simulink model "bipedal_robot_buV2_4"  (R2020b)
settings: Solver=ode23  StartTime=0.0  StopTime=Tsim  MaxStep=0.01  RelTol=1e-3  AbsTol=1e-3  EnableMultiTasking=on
undefined symbols (not defined in the file): Base, ctrl_config, ctrl_data, g, LefAnklePitch, LefAnkleRoll, LefHipPitch, LefHipRoll, LefHipYaw, LefKnee, lleg_str, RigAnklePitch, RigAnkleRoll, RigHipPitch, RigHipRoll, RigHipYaw, RigKnee, rleg_str, sim_floor, Tfil, TG_test_type, total_mass, Ts, X, Y, Z
libraries: sm_lib x53, biped_lib x34, nesl_utility x9, robotmaniplib x5, simulink x1, Contact_Forces_Lib x1
(part 2 of 3)

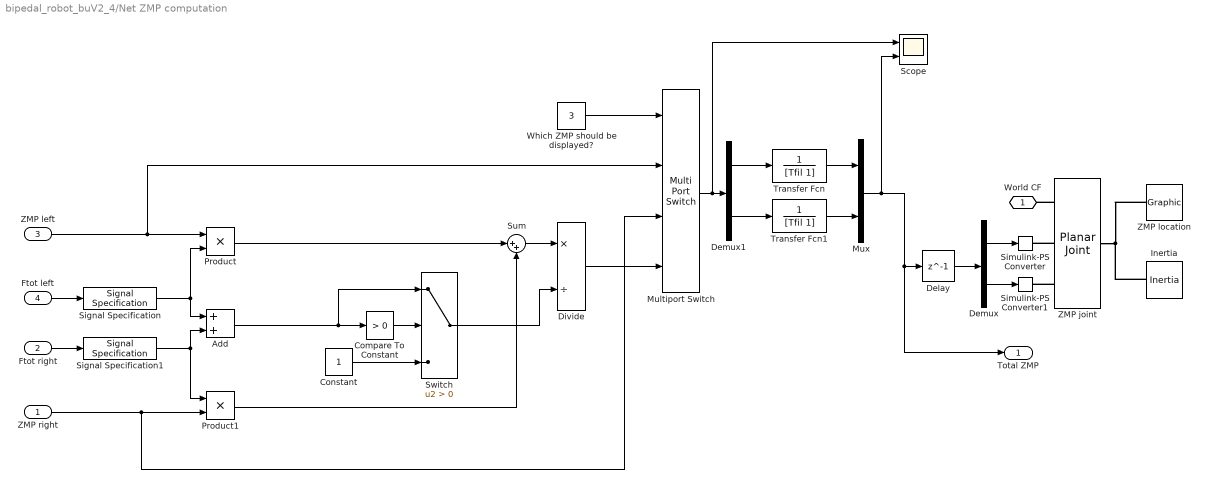
== system bipedal_robot_buV2_4/Net ZMP computation ==
  ZMP right : Inport
  Ftot right : Inport  Port=2
  ZMP left : Inport  Port=3
  Ftot left : Inport  Port=4
  Add : Sum
  Compare To Constant : simulink/Logic and Bit Operations/Compare To Constant  relop=>  const=0  OutDataTypeStr=boolean
  Constant : Constant
  Delay : Delay  DelayLength=1  InitialCondition=0  SampleTime=Ts/10
  Demux : Demux  Outputs=2
  Demux1 : Demux  Outputs=2
  Divide : Product  Inputs=*/
  Inertia : sm_lib/Body Elements/Inertia  InertiaType=Custom  Mass=10  MassUnits=g  CenterOfMass=[0 0 0]  CenterOfMassUnits=m  MomentsOfInertia=ones(3,1)*0.001  MomentsOfInertiaUnits=kg*m^2  ProductsOfInertia=[0 0 0]  ProductsOfInertiaUnits=kg*m^2  GraphicType=None  MarkerShape=Inertia  MarkerSize=20  GraphicVisPropType=SimpleVisualProperties  GraphicDiffuseColor=[0.5 0.5 0.5]  GraphicSpecularColor=[0.5 0.5 0.5 1.0]  GraphicAmbientColor=[0.15 0.15 0.15 1.0]  GraphicEmissiveColor=[0.0 0.0 0.0 1.0]  GraphicShininess=75  GraphicOpacity=1.0
  Multiport Switch : MultiPortSwitch
  Mux : Mux  Inputs=2
  Product : Product
  Product1 : Product
  Scope : Scope  NumInputPorts=2
  Signal Specification : SignalSpecification  Dimensions=1
  Signal Specification1 : SignalSpecification  Dimensions=1
  Simulink-PS Converter : nesl_utility/Simulink-PS Converter  PhysicalDomain=network_engine_domain  SubClassName=ps_input  LeftPortType=input  RightPortType=output  PseudoPeriodic=off  Frequencies=[]  NoiseDistribution=none  NoiseParameters=[]  Unit=1  AffineConversion=off  FilteringAndDerivatives=zero  SimscapeFilterOrder=1  InputFilterTimeConstant=0.001  UdotUserProvided=0
      settings: SourceProductName=Utilities
  Simulink-PS Converter1 : nesl_utility/Simulink-PS Converter  PhysicalDomain=network_engine_domain  SubClassName=ps_input  LeftPortType=input  RightPortType=output  PseudoPeriodic=off  Frequencies=[]  NoiseDistribution=none  NoiseParameters=[]  Unit=1  AffineConversion=off  FilteringAndDerivatives=zero  SimscapeFilterOrder=1  InputFilterTimeConstant=0.001  UdotUserProvided=0
      settings: SourceProductName=Utilities
  Sum : Sum  Inputs=|++
  Switch : Switch  Criteria=u2 > Threshold
  Transfer Fcn : TransferFcn  Denominator=[Tfil 1]
  Transfer Fcn1 : TransferFcn  Denominator=[Tfil 1]
  Which ZMP should be displayed? : Constant  Value=3
  ZMP joint : sm_lib/Joints/Planar Joint  JointMode=Normal  SenseConstraintForce=off  SenseConstraintForceX=off  SenseConstraintForceY=off  SenseConstraintForceZ=off  SenseConstraintTorque=off  SenseConstraintTorqueX=off  SenseConstraintTorqueY=off  SenseConstraintTorqueZ=off  SenseTotalForce=off  SenseTotalForceX=off  SenseTotalForceY=off  SenseTotalForceZ=off  SenseTotalTorque=off  SenseTotalTorqueX=off  SenseTotalTorqueY=off  SenseTotalTorqueZ=off  CompositeWrenchDir=FollowerOnBase  CompositeWrenchFrame=BaseFrame  PxEquilibriumPosition=0  PxEquilibriumPositionUnits=m  PxSpringStiffness=0  PxSpringStiffnessUnits=N/m  PxDampingCoefficient=0  PxDampingCoefficientUnits=N/(m/s)  PxTorqueActuationMode=ComputedTorque  PxMotionActuationMode=InputMotion  PxSensePosition=off  PxSenseVelocity=off  PxSenseAcceleration=off  PxSenseTorqueForce=off  PxSenseLowerLimitTorqueForce=off  PxSenseUpperLimitTorqueForce=off  PxLowerLimitSpecify=off  PxLowerLimitBound=-1  PxLowerLimitBoundUnits=m  PxLowerLimitStiffness=1e6  PxLowerLimitStiffnessUnits=N/m  PxLowerLimitDamping=1e3  PxLowerLimitDampingUnits=N/(m/s)  PxLowerLimitTransitionRegionWidth=1e-4  PxLowerLimitTransitionRegionWidthUnits=m  PxUpperLimitSpecify=off  PxUpperLimitBound=1  PxUpperLimitBoundUnits=m  PxUpperLimitStiffness=1e6  PxUpperLimitStiffnessUnits=N/m  PxUpperLimitDamping=1e3  PxUpperLimitDampingUnits=N/(m/s)  PxUpperLimitTransitionRegionWidth=1e-4  PxUpperLimitTransitionRegionWidthUnits=m  PxPositionTargetSpecify=off  PxPositionTargetPriority=High  PxPositionTargetValue=0  PxPositionTargetValueUnits=m  PxVelocityTargetSpecify=off  PxVelocityTargetPriority=High  PxVelocityTargetValue=0  PxVelocityTargetValueUnits=m/s  PyEquilibriumPosition=0  PyEquilibriumPositionUnits=m  PySpringStiffness=0  PySpringStiffnessUnits=N/m  PyDampingCoefficient=0  PyDampingCoefficientUnits=N/(m/s)  PyTorqueActuationMode=ComputedTorque  PyMotionActuationMode=InputMotion  PySensePosition=off  PySenseVelocity=off  PySenseAcceleration=off  PySenseTorqueForce=off  PySenseLowerLimitTorqueForce=off  PySenseUpperLimitTorqueForce=off  PyLowerLimitSpecify=off  PyLowerLimitBound=-1  PyLowerLimitBoundUnits=m  PyLowerLimitStiffness=1e6  PyLowerLimitStiffnessUnits=N/m  PyLowerLimitDamping=1e3  PyLowerLimitDampingUnits=N/(m/s)  PyLowerLimitTransitionRegionWidth=1e-4  PyLowerLimitTransitionRegionWidthUnits=m  PyUpperLimitSpecify=off  PyUpperLimitBound=1  PyUpperLimitBoundUnits=m  PyUpperLimitStiffness=1e6  PyUpperLimitStiffnessUnits=N/m  PyUpperLimitDamping=1e3  PyUpperLimitDampingUnits=N/(m/s)  PyUpperLimitTransitionRegionWidth=1e-4  PyUpperLimitTransitionRegionWidthUnits=m  PyPositionTargetSpecify=off  PyPositionTargetPriority=High  PyPositionTargetValue=0  PyPositionTargetValueUnits=m  PyVelocityTargetSpecify=off  PyVelocityTargetPriority=High  PyVelocityTargetValue=0  PyVelocityTargetValueUnits=m/s  RzEquilibriumPosition=0  RzEquilibriumPositionUnits=deg  RzSpringStiffness=0  RzSpringStiffnessUnits=N*m/deg  RzDampingCoefficient=0  RzDampingCoefficientUnits=N*m/(deg/s)  RzTorqueActuationMode=NoTorque  RzMotionActuationMode=ComputedMotion  RzSensePosition=off  RzSenseVelocity=off  RzSenseAcceleration=off  RzSenseTorqueForce=off  RzSenseLowerLimitTorqueForce=off  RzSenseUpperLimitTorqueForce=off  RzLowerLimitSpecify=off  RzLowerLimitBound=-90  RzLowerLimitBoundUnits=deg  RzLowerLimitStiffness=1e4  RzLowerLimitStiffnessUnits=N*m/deg  RzLowerLimitDamping=10  RzLowerLimitDampingUnits=N*m/(deg/s)  RzLowerLimitTransitionRegionWidth=0.1  RzLowerLimitTransitionRegionWidthUnits=deg  RzUpperLimitSpecify=off  RzUpperLimitBound=90  RzUpperLimitBoundUnits=deg  RzUpperLimitStiffness=1e4  RzUpperLimitStiffnessUnits=N*m/deg  RzUpperLimitDamping=10  RzUpperLimitDampingUnits=N*m/(deg/s)  RzUpperLimitTransitionRegionWidth=0.1  RzUpperLimitTransitionRegionWidthUnits=deg  RzPositionTargetSpecify=off  RzPositionTargetPriority=High  RzPositionTargetValue=0  RzPositionTargetValueUnits=deg  RzVelocityTargetSpecify=off  RzVelocityTargetPriority=High  RzVelocityTargetValue=0  RzVelocityTargetValueUnits=deg/s
  ZMP location : sm_lib/Body Elements/Graphic  GraphicType=Marker  MarkerShape=Frame  MarkerSize=30  GraphicVisPropType=SimpleVisualProperties  GraphicDiffuseColor=[0.0 1.0 0.2]  GraphicSpecularColor=[0.5 0.5 0.5 1.0]  GraphicAmbientColor=[0.15 0.15 0.15 1.0]  GraphicEmissiveColor=[0.0 0.0 0.0 1.0]  GraphicShininess=75  GraphicOpacity=1.0
  World CF : PMIOPort  Side=Left
  Total ZMP : Outport
  wires:
  ZMP left/1 -> Product/1, Multiport Switch/2
  Signal Specification/1 -> Product/2, Add/1
  Signal Specification1/1 -> Product1/1, Add/2
  ZMP right/1 -> Multiport Switch/3, Product1/2
  Product/1 -> Sum/1
  Product1/1 -> Sum/2
  Sum/1 -> Divide/1
  Add/1 -> Compare To Constant/1, Switch/1
  Mux/1 -> Total ZMP/1, Delay/1, Scope/2
  Demux/1 -> Simulink-PS Converter/1
  Demux/2 -> Simulink-PS Converter1/1
  Compare To Constant/1 -> Switch/2
  Constant/1 -> Switch/3
  Switch/1 -> Divide/2
  Ftot left/1 -> Signal Specification/1
  Ftot right/1 -> Signal Specification1/1
  Delay/1 -> Demux/1
  Which ZMP should be displayed?/1 -> Multiport Switch/1
  Divide/1 -> Multiport Switch/4
  Demux1/1 -> Transfer Fcn/1
  Demux1/2 -> Transfer Fcn1/1
  Multiport Switch/1 -> Scope/1, Demux1/1
  Transfer Fcn1/1 -> Mux/2
  Transfer Fcn/1 -> Mux/1
  connections:
  ZMP joint/LConn1 -- World CF/RConn1
  ZMP location/RConn1 -- Inertia/RConn1 -- ZMP joint/RConn1
  ZMP joint/LConn2 -- Simulink-PS Converter/RConn1
  ZMP joint/LConn3 -- Simulink-PS Converter1/RConn1

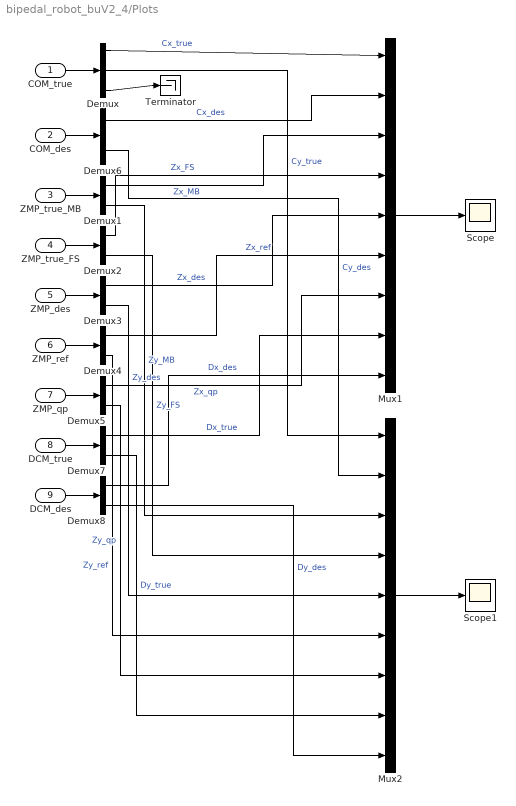
== system bipedal_robot_buV2_4/Plots ==
  COM_true : Inport
  COM_des : Inport  Port=2
  ZMP_true_MB : Inport  Port=3
  ZMP_true_FS : Inport  Port=4
  ZMP_des : Inport  Port=5
  ZMP_ref : Inport  Port=6
  ZMP_qp : Inport  Port=7
  DCM_true : Inport  Port=8
  DCM_des : Inport  Port=9
  Demux : Demux  Outputs=3
  Demux{1..8} (8 alike) : Demux  Outputs=2
  Mux1 : Mux  Inputs=9
  Mux2 : Mux  Inputs=9
  Scope : Scope
  Scope1 : Scope
  Terminator : Terminator
  wires:
  ZMP_true_MB/1 -> Demux1/1
  ZMP_true_FS/1 -> Demux2/1
  ZMP_des/1 -> Demux3/1
  ZMP_ref/1 -> Demux4/1
  ZMP_qp/1 -> Demux5/1
  COM_true/1 -> Demux/1
  DCM_true/1 -> Demux7/1
  DCM_des/1 -> Demux8/1
  Demux/1 -> Mux1/1  "Cx_true"
  Demux6/1 -> Mux1/2  "Cx_des"
  Demux1/1 -> Mux1/3  "Zx_MB"
  Demux2/1 -> Mux1/4  "Zx_FS"
  Demux3/1 -> Mux1/5  "Zx_des"
  Demux4/1 -> Mux1/6  "Zx_ref"
  Demux5/1 -> Mux1/7  "Zx_qp"
  Demux7/1 -> Mux1/8  "Dx_true"
  Demux8/1 -> Mux1/9  "Dx_des"
  Demux/2 -> Mux2/1  "Cy_true"
  Demux1/2 -> Mux2/3  "Zy_MB"
  Demux2/2 -> Mux2/4  "Zy_FS"
  Demux3/2 -> Mux2/5  "Zy_des"
  Demux4/2 -> Mux2/6  "Zy_ref"
  Demux5/2 -> Mux2/7  "Zy_qp"
  Demux7/2 -> Mux2/8  "Dy_true"
  Demux8/2 -> Mux2/9  "Dy_des"
  Demux6/2 -> Mux2/2  "Cy_des"
  Demux/3 -> Terminator/1
  Mux1/1 -> Scope/1
  Mux2/1 -> Scope1/1
  COM_des/1 -> Demux6/1

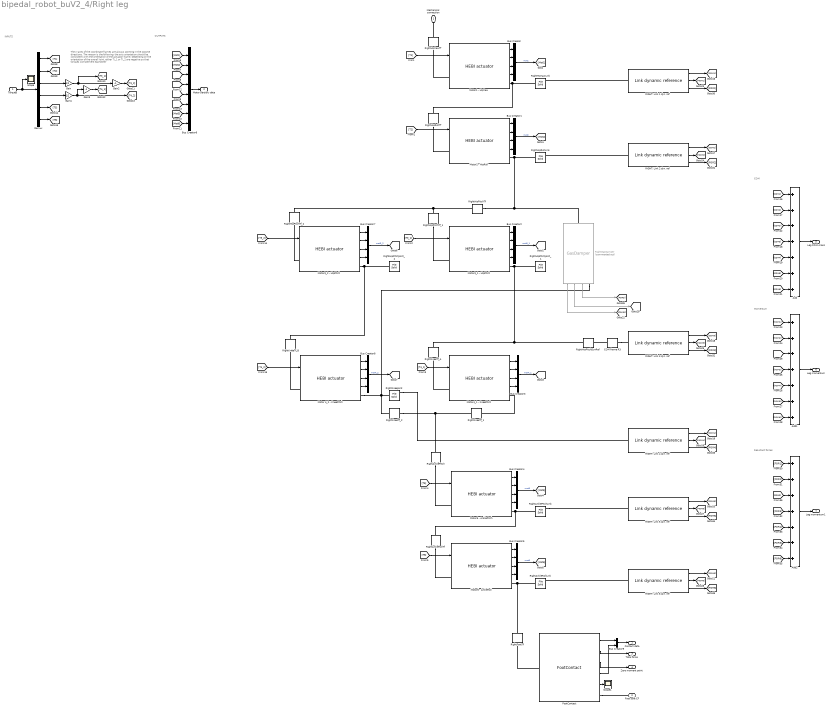
== system bipedal_robot_buV2_4/Right leg ==
  note: OUTPUTS
  note: INPUTS
  note: The z-axes of the coordinate frames are always pointing in the
      | oposite directions. The reason is the following: the axis orientation
      | should be consistent with the orientation of the actuator frame. Depending on the orientation of the overall joint, either Ti_1 or Ti_2
      | are negative so that torques complement eachother
  note: Resultant forces
  note: Momentum
  note: COM
  Torques : Inport
  Add : Sum  Inputs=7
  Add1 : Sum  Inputs=7
  Add2 : Sum  Inputs=7
  Bus Creator{,1..5,7..8} (8 alike) : BusCreator  Inputs=4
  Bus Creator6 : BusCreator  Inputs=8  OutDataTypeStr=Bus: leg_str_bus
  Bus Creator9 : BusCreator  Inputs=2
  COM frame R3 : sm_lib/Frames and Transforms/Rigid Transform  TranslationMethod=Cartesian  TranslationStandardOffset=0  TranslationLengthUnit=m  TranslationStandardAxis=+Z  TranslationCartesianOffset=RigHipPitch.body.com  TranslationROffset=0  TranslationROffsetUnits=m  TranslationZOffset=0  TranslationZOffsetUnits=m  TranslationThetaOffset=0  TranslationThetaOffsetUnits=deg  RotationMethod=None  RotationAngleUnits=deg  RotationStandardAxis=+Z  RotationAngle=0.0  RotationArbitraryAxis=[0 0 1]  FollAlignAxisA=+X  BaseAlignAxisA=+Y  FollAlignAxisB=+Y  BaseAlignAxisB=+Z  RotationSequenceAxes=FollowerAxes  RotationSequence=XYX  RotationSequenceAngles=[0 0 0]  RotationSequenceAnglesUnits=deg  RotationMatrix=[1 0 0; 0 1 0; 0 0 1]
  Demux : Demux  Outputs=6
  FootContact : biped_lib/FootContact  SystemSampleTime=-1  VariantActivationTime=update diagram  Latency=0  AutoFrameSizeCalculation=off
  Gain : Gain  Gain=1/2
  Gain1 : Gain  Gain=1/2
  Gain2 : Gain  Gain=-1
  Gain3 : Gain  Gain=-1
  Motor 4_2 - KneePitch : biped_lib/HEBI actuator  Tmax=motor.X8.v16.Tmax  qinit=RigKnee.qinit_2  IMU=RigKnee.IMU_2
  Motor1 - HipYaw : biped_lib/HEBI actuator  Tmax=motor.X8.v16.Tmax  qinit=RigHipYaw.qinit  IMU=RigHipYaw.IMU
  Motor2 - HipRoll : biped_lib/HEBI actuator  Tmax=motor.X8.v16.Tmax  qinit=RigHipRoll.qinit  IMU=RigHipRoll.IMU
  Motor3_1 - HipPitch : biped_lib/HEBI actuator  Tmax=motor.X8.v16.Tmax  qinit=RigHipPitch.qinit_1  IMU=RigHipPitch.IMU_1
  Motor3_2 - HipPitch : biped_lib/HEBI actuator  Tmax=motor.X8.v16.Tmax  qinit=RigHipPitch.qinit_2  IMU=RigHipPitch.IMU_2
  Motor4_1 - KneePitch : biped_lib/HEBI actuator  Tmax=motor.X8.v16.Tmax  qinit=RigKnee.qinit_1  IMU=RigKnee.IMU_1
  Motor5 - AnklePitch : biped_lib/HEBI actuator  Tmax=motor.X8.v16.Tmax  qinit=RigAnklePitch.qinit  IMU=RigAnklePitch.IMU
  Motor6 - AnkleRoll : biped_lib/HEBI actuator  Tmax=motor.X8.v16.Tmax  qinit=RigAnkleRoll.qinit  IMU=RigAnkleRoll.IMU
  RIGHT: Link 1 dyn. ref : biped_lib/Link dynamic reference  M=RigHipYaw.body.mass  I=RigHipYaw.body.inertia
  RIGHT: Link 2 dyn. ref : biped_lib/Link dynamic reference  M=RigHipRoll.body.mass  I=RigHipRoll.body.inertia
  RIGHT: Link 3 dyn. ref : biped_lib/Link dynamic reference  M=RigHipPitch.body.mass  I=RigHipPitch.body.inertia
  RIGHT: Link 4 dyn. ref : biped_lib/Link dynamic reference  M=RigKnee.body.mass  I=RigKnee.body.inertia
  RIGHT: Link 5 dyn. ref : biped_lib/Link dynamic reference  M=RigAnklePitch.body.mass  I=RigAnklePitch.body.inertia
  RIGHT: Link 6 dyn. ref : biped_lib/Link dynamic reference  M=RigAnkleRoll.body.mass  I=RigAnkleRoll.body.inertia
  RightAnklePitch : sm_lib/Frames and Transforms/Rigid Transform  TranslationMethod=Cartesian  TranslationStandardOffset=0  TranslationLengthUnit=m  TranslationStandardAxis=+Z  TranslationCartesianOffset=RigAnklePitch.pos  TranslationROffset=0  TranslationROffsetUnits=m  TranslationZOffset=0  TranslationZOffsetUnits=m  TranslationThetaOffset=0  TranslationThetaOffsetUnits=deg  RotationMethod=RotationSequence  RotationAngleUnits=deg  RotationStandardAxis=+Z  RotationAngle=0.0  RotationArbitraryAxis=[0 0 1]  FollAlignAxisA=+X  BaseAlignAxisA=+Y  FollAlignAxisB=+Y  BaseAlignAxisB=+Z  RotationSequenceAxes=FollowerAxes  RotationSequence=XYZ  RotationSequenceAngles=RigAnklePitch.rot  RotationSequenceAnglesUnits=rad  RotationMatrix=[1 0 0; 0 1 0; 0 0 1]
  RightAnklePitchLink : sm_lib/Body Elements/File Solid  ExtGeomFileName=Link5R_LR.stl  UnitType=Custom  ExtGeomFileUnits=mm  StepReaderType=HEX  ExportConvexHullGeometry=on  InertiaType=CalculateFromGeometry  Mass=RigAnklePitch.body.mass  MassUnits=kg  CenterOfMass=[0 0 0]  CenterOfMassUnits=m  MomentsOfInertia=[1 1 1]  MomentsOfInertiaUnits=kg*m^2  ProductsOfInertia=[0 0 0]  ProductsOfInertiaUnits=kg*m^2  BasedOnType=Mass  Density=1000  DensityUnits=kg/m^3  DoExposeReferenceFrame=on  SerializedFrames=<Frames><Frame><Id>Frame1</Id><Value><Name>COM</Name><Origin><Source>CenterOfMassFrame</Source><FeatureName></FeatureName></Origin><PrimaryAxis><DefinedDirection>+Z</DefinedDirection><Source>ReferenceFrame</Source><SourceDirection>+Z</SourceDirection><FeatureName></FeatureName></PrimaryAxis><SecondaryAxis><DefinedDirection>+X</DefinedDirection><Source>ReferenceFrame</Source><SourceDirection>+X</SourceDirection><FeatureName></FeatureName></SecondaryAxis></Value></Frame></Frames>  GraphicType=FromGeometry  MarkerShape=Sphere  MarkerSize=10  GraphicVisPropType=SimpleVisualProperties  GraphicDiffuseColor=[0.5 0.5 0.5]  GraphicSpecularColor=[0.5 0.5 0.5 1.0]  GraphicAmbientColor=[0.15 0.15 0.15 1.0]  GraphicEmissiveColor=[0.0 0.0 0.0 1.0]  GraphicShininess=75  GraphicOpacity=1.0
  RightAnkleRollLink : sm_lib/Body Elements/File Solid  ExtGeomFileName=Link6_LR.stl  UnitType=Custom  ExtGeomFileUnits=mm  StepReaderType=HEX  ExportConvexHullGeometry=on  InertiaType=CalculateFromGeometry  Mass=RigAnkleRoll.body.mass  MassUnits=kg  CenterOfMass=[0 0 0]  CenterOfMassUnits=m  MomentsOfInertia=[1 1 1]  MomentsOfInertiaUnits=kg*m^2  ProductsOfInertia=[0 0 0]  ProductsOfInertiaUnits=kg*m^2  BasedOnType=Mass  Density=1000  DensityUnits=kg/m^3  DoExposeReferenceFrame=on  SerializedFrames=<Frames><Frame><Id>Frame1</Id><Value><Name>COM</Name><Origin><Source>CenterOfMassFrame</Source><FeatureName></FeatureName></Origin><PrimaryAxis><DefinedDirection>+Z</DefinedDirection><Source>ReferenceFrame</Source><SourceDirection>+Z</SourceDirection><FeatureName></FeatureName></PrimaryAxis><SecondaryAxis><DefinedDirection>+X</DefinedDirection><Source>ReferenceFrame</Source><SourceDirection>+X</SourceDirection><FeatureName></FeatureName></SecondaryAxis></Value></Frame></Frames>  GraphicType=FromGeometry  MarkerShape=Sphere  MarkerSize=10  GraphicVisPropType=SimpleVisualProperties  GraphicDiffuseColor=[0.5 0.5 0.5]  GraphicSpecularColor=[0.5 0.5 0.5 1.0]  GraphicAmbientColor=[0.15 0.15 0.15 1.0]  GraphicEmissiveColor=[0.0 0.0 0.0 1.0]  GraphicShininess=75  GraphicOpacity=1.0
  RightAnkleRollTf : sm_lib/Frames and Transforms/Rigid Transform  TranslationMethod=Cartesian  TranslationStandardOffset=0  TranslationLengthUnit=m  TranslationStandardAxis=+Z  TranslationCartesianOffset=RigAnkleRoll.pos  TranslationROffset=0  TranslationROffsetUnits=m  TranslationZOffset=0  TranslationZOffsetUnits=m  TranslationThetaOffset=0  TranslationThetaOffsetUnits=deg  RotationMethod=RotationSequence  RotationAngleUnits=deg  RotationStandardAxis=+Z  RotationAngle=0.0  RotationArbitraryAxis=[0 0 1]  FollAlignAxisA=+Z  BaseAlignAxisA=+X  FollAlignAxisB=+Y  BaseAlignAxisB=+Y  RotationSequenceAxes=FollowerAxes  RotationSequence=XYZ  RotationSequenceAngles=RigAnkleRoll.rot  RotationSequenceAnglesUnits=rad  RotationMatrix=[1 0 0; 0 1 0; 0 0 1]
  RightFootTf : sm_lib/Frames and Transforms/Rigid Transform  TranslationMethod=Cartesian  TranslationStandardOffset=0  TranslationLengthUnit=m  TranslationStandardAxis=+Z  TranslationCartesianOffset=RigFoot.pos  TranslationROffset=0  TranslationROffsetUnits=m  TranslationZOffset=0  TranslationZOffsetUnits=m  TranslationThetaOffset=0  TranslationThetaOffsetUnits=deg  RotationMethod=RotationSequence  RotationAngleUnits=deg  RotationStandardAxis=+Z  RotationAngle=0.0  RotationArbitraryAxis=[0 0 1]  FollAlignAxisA=+Z  BaseAlignAxisA=+Y  FollAlignAxisB=+X  BaseAlignAxisB=+X  RotationSequenceAxes=FollowerAxes  RotationSequence=XYZ  RotationSequenceAngles=RigFoot.rot  RotationSequenceAnglesUnits=rad  RotationMatrix=[1 0 0; 0 1 0; 0 0 1]
  RightGasDamper : biped_lib/GasDamper  Commented=on  mech=RigDamper
  RightHipPitchDynRef : sm_lib/Frames and Transforms/Rigid Transform  TranslationMethod=Cartesian  TranslationStandardOffset=0  TranslationLengthUnit=m  TranslationStandardAxis=+Z  TranslationCartesianOffset=-RigHipPitch.pos_1  TranslationROffset=0  TranslationROffsetUnits=m  TranslationZOffset=0  TranslationZOffsetUnits=m  TranslationThetaOffset=0  TranslationThetaOffsetUnits=deg  RotationMethod=None  RotationAngleUnits=deg  RotationStandardAxis=+Z  RotationAngle=0.0  RotationArbitraryAxis=[0 0 1]  FollAlignAxisA=+X  BaseAlignAxisA=+Y  FollAlignAxisB=+Y  BaseAlignAxisB=+Z  RotationSequenceAxes=FollowerAxes  RotationSequence=XYX  RotationSequenceAngles=[0 0 0]  RotationSequenceAnglesUnits=deg  RotationMatrix=[1 0 0; 0 1 0; 0 0 1]
  RightHipPitchJoint_1 : sm_lib/Body Elements/File Solid  ExtGeomFileName=Link3_LR.stl  UnitType=Custom  ExtGeomFileUnits=mm  StepReaderType=HEX  ExportConvexHullGeometry=on  InertiaType=CalculateFromGeometry  Mass=RigHipPitch.body.mass  MassUnits=kg  CenterOfMass=[0 0 0]  CenterOfMassUnits=m  MomentsOfInertia=[1 1 1]  MomentsOfInertiaUnits=kg*m^2  ProductsOfInertia=[0 0 0]  ProductsOfInertiaUnits=kg*m^2  BasedOnType=Mass  Density=1000  DensityUnits=kg/m^3  DoExposeReferenceFrame=on  SerializedFrames=<Frames/>  GraphicType=FromGeometry  MarkerShape=Sphere  MarkerSize=10  GraphicVisPropType=SimpleVisualProperties  GraphicDiffuseColor=[0.5 0.5 0.5]  GraphicSpecularColor=[0.5 0.5 0.5 1.0]  GraphicAmbientColor=[0.15 0.15 0.15 1.0]  GraphicEmissiveColor=[0.0 0.0 0.0 1.0]  GraphicShininess=75  GraphicOpacity=1.0
  RightHipPitchJoint_2 : sm_lib/Body Elements/File Solid  ExtGeomFileName=Link3_LR.stl  UnitType=Custom  ExtGeomFileUnits=mm  StepReaderType=HEX  ExportConvexHullGeometry=on  InertiaType=CalculateFromGeometry  Mass=RigHipPitch.body.mass  MassUnits=kg  CenterOfMass=[0 0 0]  CenterOfMassUnits=m  MomentsOfInertia=[1 1 1]  MomentsOfInertiaUnits=kg*m^2  ProductsOfInertia=[0 0 0]  ProductsOfInertiaUnits=kg*m^2  BasedOnType=Mass  Density=1000  DensityUnits=kg/m^3  DoExposeReferenceFrame=on  SerializedFrames=<Frames/>  GraphicType=FromGeometry  MarkerShape=Sphere  MarkerSize=10  GraphicVisPropType=SimpleVisualProperties  GraphicDiffuseColor=[0.5 0.5 0.5]  GraphicSpecularColor=[0.5 0.5 0.5 1.0]  GraphicAmbientColor=[0.15 0.15 0.15 1.0]  GraphicEmissiveColor=[0.0 0.0 0.0 1.0]  GraphicShininess=75  GraphicOpacity=1.0
  RightHipPitchTf : sm_lib/Frames and Transforms/Rigid Transform  TranslationMethod=Cartesian  TranslationStandardOffset=0  TranslationLengthUnit=m  TranslationStandardAxis=+Z  TranslationCartesianOffset=RigHipPitch.pos  TranslationROffset=0  TranslationROffsetUnits=m  TranslationZOffset=0  TranslationZOffsetUnits=m  TranslationThetaOffset=0  TranslationThetaOffsetUnits=deg  RotationMethod=RotationSequence  RotationAngleUnits=deg  RotationStandardAxis=+Z  RotationAngle=0.0  RotationArbitraryAxis=[0 0 1]  FollAlignAxisA=+Z  BaseAlignAxisA=-X  FollAlignAxisB=+Y  BaseAlignAxisB=+Y  RotationSequenceAxes=FollowerAxes  RotationSequence=XYX  RotationSequenceAngles=RigHipPitch.rot  RotationSequenceAnglesUnits=rad  RotationMatrix=[1 0 0; 0 1 0; 0 0 1]
  RightHipPitchTf_1 : sm_lib/Frames and Transforms/Rigid Transform  TranslationMethod=Cartesian  TranslationStandardOffset=0  TranslationLengthUnit=m  TranslationStandardAxis=+Z  TranslationCartesianOffset=RigHipPitch.pos_1  TranslationROffset=0  TranslationROffsetUnits=m  TranslationZOffset=0  TranslationZOffsetUnits=m  TranslationThetaOffset=0  TranslationThetaOffsetUnits=deg  RotationMethod=RotationSequence  RotationAngleUnits=deg  RotationStandardAxis=+Z  RotationAngle=0.0  RotationArbitraryAxis=[0 0 1]  FollAlignAxisA=+X  BaseAlignAxisA=+Y  FollAlignAxisB=+Y  BaseAlignAxisB=+Z  RotationSequenceAxes=FollowerAxes  RotationSequence=XYZ  RotationSequenceAngles=RigHipPitch.rot_1  RotationSequenceAnglesUnits=rad  RotationMatrix=[1 0 0; 0 1 0; 0 0 1]
  RightHipPitchTf_2 : sm_lib/Frames and Transforms/Rigid Transform  TranslationMethod=Cartesian  TranslationStandardOffset=0  TranslationLengthUnit=m  TranslationStandardAxis=+Z  TranslationCartesianOffset=RigHipPitch.pos_2  TranslationROffset=0  TranslationROffsetUnits=m  TranslationZOffset=0  TranslationZOffsetUnits=m  TranslationThetaOffset=0  TranslationThetaOffsetUnits=deg  RotationMethod=RotationSequence  RotationAngleUnits=deg  RotationStandardAxis=+Z  RotationAngle=0.0  RotationArbitraryAxis=[0 0 1]  FollAlignAxisA=+X  BaseAlignAxisA=+Y  FollAlignAxisB=+Y  BaseAlignAxisB=+Z  RotationSequenceAxes=FollowerAxes  RotationSequence=XYZ  RotationSequenceAngles=RigHipPitch.rot_2  RotationSequenceAnglesUnits=rad  RotationMatrix=[1 0 0; 0 1 0; 0 0 1]
  RightHipRollLink : sm_lib/Body Elements/File Solid  ExtGeomFileName=Link2_LR.stl  UnitType=Custom  ExtGeomFileUnits=mm  StepReaderType=HEX  ExportConvexHullGeometry=on  InertiaType=CalculateFromGeometry  Mass=RigHipRoll.body.mass  MassUnits=kg  CenterOfMass=[0 0 0]  CenterOfMassUnits=m  MomentsOfInertia=[1 1 1]  MomentsOfInertiaUnits=kg*m^2  ProductsOfInertia=[0 0 0]  ProductsOfInertiaUnits=kg*m^2  BasedOnType=Mass  Density=1000  DensityUnits=kg/m^3  DoExposeReferenceFrame=on  SerializedFrames=<Frames><Frame><Id>Frame1</Id><Value><Name>COM</Name><Origin><Source>CenterOfMassFrame</Source><FeatureName></FeatureName></Origin><PrimaryAxis><DefinedDirection>+Z</DefinedDirection><Source>ReferenceFrame</Source><SourceDirection>+Z</SourceDirection><FeatureName></FeatureName></PrimaryAxis><SecondaryAxis><DefinedDirection>+X</DefinedDirection><Source>ReferenceFrame</Source><SourceDirection>+X</SourceDirection><FeatureName></FeatureName></SecondaryAxis></Value></Frame></Frames>  GraphicType=FromGeometry  MarkerShape=Sphere  MarkerSize=10  GraphicVisPropType=SimpleVisualProperties  GraphicDiffuseColor=[0.5 0.5 0.5]  GraphicSpecularColor=[0.5 0.5 0.5 1.0]  GraphicAmbientColor=[0.15 0.15 0.15 1.0]  GraphicEmissiveColor=[0.0 0.0 0.0 1.0]  GraphicShininess=75  GraphicOpacity=1.0
  RightHipRollTf : sm_lib/Frames and Transforms/Rigid Transform  TranslationMethod=Cartesian  TranslationStandardOffset=0  TranslationLengthUnit=m  TranslationStandardAxis=+Z  TranslationCartesianOffset=RigHipRoll.pos  TranslationROffset=0  TranslationROffsetUnits=m  TranslationZOffset=0  TranslationZOffsetUnits=m  TranslationThetaOffset=0  TranslationThetaOffsetUnits=deg  RotationMethod=RotationSequence  RotationAngleUnits=deg  RotationStandardAxis=+Z  RotationAngle=0.0  RotationArbitraryAxis=[0 0 1]  FollAlignAxisA=+Z  BaseAlignAxisA=+Y  FollAlignAxisB=+X  BaseAlignAxisB=+X  RotationSequenceAxes=FollowerAxes  RotationSequence=XYZ  RotationSequenceAngles=RigHipRoll.rot  RotationSequenceAnglesUnits=rad  RotationMatrix=[1 0 0; 0 1 0; 0 0 1]
  RightHipYawLink : sm_lib/Body Elements/File Solid  ExtGeomFileName=Link1R_LR.stl  UnitType=Custom  ExtGeomFileUnits=mm  StepReaderType=HEX  ExportConvexHullGeometry=on  InertiaType=CalculateFromGeometry  Mass=RigHipYaw.body.mass  MassUnits=kg  CenterOfMass=[0 0 0]  CenterOfMassUnits=m  MomentsOfInertia=[1 1 1]  MomentsOfInertiaUnits=kg*m^2  ProductsOfInertia=[0 0 0]  ProductsOfInertiaUnits=kg*m^2  BasedOnType=Mass  Density=1000  DensityUnits=kg/m^3  DoExposeReferenceFrame=on  SerializedFrames=<Frames><Frame><Id>Frame1</Id><Value><Name>COM</Name><Origin><Source>CenterOfMassFrame</Source><FeatureName></FeatureName></Origin><PrimaryAxis><DefinedDirection>+Z</DefinedDirection><Source>ReferenceFrame</Source><SourceDirection>+Z</SourceDirection><FeatureName></FeatureName></PrimaryAxis><SecondaryAxis><DefinedDirection>+X</DefinedDirection><Source>ReferenceFrame</Source><SourceDirection>+X</SourceDirection><FeatureName></FeatureName></SecondaryAxis></Value></Frame></Frames>  GraphicType=FromGeometry  MarkerShape=Sphere  MarkerSize=10  GraphicVisPropType=SimpleVisualProperties  GraphicDiffuseColor=[0.5 0.5 0.5]  GraphicSpecularColor=[0.5 0.5 0.5 1.0]  GraphicAmbientColor=[0.15 0.15 0.15 1.0]  GraphicEmissiveColor=[0.0 0.0 0.0 1.0]  GraphicShininess=75  GraphicOpacity=1.0
  RightHipYawTf : sm_lib/Frames and Transforms/Rigid Transform  TranslationMethod=Cartesian  TranslationStandardOffset=0  TranslationLengthUnit=m  TranslationStandardAxis=+Z  TranslationCartesianOffset=RigHipYaw.pos  TranslationROffset=0  TranslationROffsetUnits=m  TranslationZOffset=0  TranslationZOffsetUnits=m  TranslationThetaOffset=0  TranslationThetaOffsetUnits=deg  RotationMethod=RotationSequence  RotationAngleUnits=deg  RotationStandardAxis=+Z  RotationAngle=0.0  RotationArbitraryAxis=[0 0 1]  FollAlignAxisA=+X  BaseAlignAxisA=+Y  FollAlignAxisB=+Y  BaseAlignAxisB=+Z  RotationSequenceAxes=FollowerAxes  RotationSequence=XYZ  RotationSequenceAngles=RigHipYaw.rot  RotationSequenceAnglesUnits=rad  RotationMatrix=[1 0 0; 0 1 0; 0 0 1]
  RightKneeJoint : sm_lib/Body Elements/File Solid  ExtGeomFileName=Link4_LR.stl  UnitType=Custom  ExtGeomFileUnits=mm  StepReaderType=HEX  ExportConvexHullGeometry=on  InertiaType=CalculateFromGeometry  Mass=LefKnee.body.mass  MassUnits=kg  CenterOfMass=[0 0 0]  CenterOfMassUnits=m  MomentsOfInertia=[1 1 1]  MomentsOfInertiaUnits=kg*m^2  ProductsOfInertia=[0 0 0]  ProductsOfInertiaUnits=kg*m^2  BasedOnType=Mass  Density=1000  DensityUnits=kg/m^3  DoExposeReferenceFrame=on  SerializedFrames=<Frames><Frame><Id>Frame1</Id><Value><Name>COM</Name><Origin><Source>CenterOfMassFrame</Source><FeatureName></FeatureName></Origin><PrimaryAxis><DefinedDirection>+Z</DefinedDirection><Source>ReferenceFrame</Source><SourceDirection>+Z</SourceDirection><FeatureName></FeatureName></PrimaryAxis><SecondaryAxis><DefinedDirection>+X</DefinedDirection><Source>ReferenceFrame</Source><SourceDirection>+X</SourceDirection><FeatureName></FeatureName></SecondaryAxis></Value></Frame></Frames>  GraphicType=FromGeometry  MarkerShape=Sphere  MarkerSize=10  GraphicVisPropType=SimpleVisualProperties  GraphicDiffuseColor=[0.5 0.5 0.5]  GraphicSpecularColor=[0.5 0.5 0.5 1.0]  GraphicAmbientColor=[0.15 0.15 0.15 1.0]  GraphicEmissiveColor=[0.0 0.0 0.0 1.0]  GraphicShininess=75  GraphicOpacity=1.0
  RightKneeTf_1 : sm_lib/Frames and Transforms/Rigid Transform  TranslationMethod=Cartesian  TranslationStandardOffset=0  TranslationLengthUnit=m  TranslationStandardAxis=+Z  TranslationCartesianOffset=RigKnee.pos_1  TranslationROffset=0  TranslationROffsetUnits=m  TranslationZOffset=0  TranslationZOffsetUnits=m  TranslationThetaOffset=0  TranslationThetaOffsetUnits=deg  RotationMethod=RotationSequence  RotationAngleUnits=deg  RotationStandardAxis=+Z  RotationAngle=0.0  RotationArbitraryAxis=[0 0 1]  FollAlignAxisA=+X  BaseAlignAxisA=+Y  FollAlignAxisB=+Y  BaseAlignAxisB=+Z  RotationSequenceAxes=FollowerAxes  RotationSequence=XYZ  RotationSequenceAngles=RigKnee.rot_1  RotationSequenceAnglesUnits=rad  RotationMatrix=[1 0 0; 0 1 0; 0 0 1]
  RightKneeTf_2 : sm_lib/Frames and Transforms/Rigid Transform  TranslationMethod=Cartesian  TranslationStandardOffset=0  TranslationLengthUnit=m  TranslationStandardAxis=+Z  TranslationCartesianOffset=RigKnee.pos_2  TranslationROffset=0  TranslationROffsetUnits=m  TranslationZOffset=0  TranslationZOffsetUnits=m  TranslationThetaOffset=0  TranslationThetaOffsetUnits=deg  RotationMethod=RotationSequence  RotationAngleUnits=deg  RotationStandardAxis=+Z  RotationAngle=0.0  RotationArbitraryAxis=[0 0 1]  FollAlignAxisA=+X  BaseAlignAxisA=+Y  FollAlignAxisB=+Y  BaseAlignAxisB=+Z  RotationSequenceAxes=FollowerAxes  RotationSequence=XYZ  RotationSequenceAngles=RigKnee.rot_2  RotationSequenceAnglesUnits=rad  RotationMatrix=[1 0 0; 0 1 0; 0 0 1]
  RightKneeTf_A : sm_lib/Frames and Transforms/Rigid Transform  TranslationMethod=Cartesian  TranslationStandardOffset=0  TranslationLengthUnit=m  TranslationStandardAxis=+Z  TranslationCartesianOffset=RigKnee.pos  TranslationROffset=0  TranslationROffsetUnits=m  TranslationZOffset=0  TranslationZOffsetUnits=m  TranslationThetaOffset=0  TranslationThetaOffsetUnits=deg  RotationMethod=RotationSequence  RotationAngleUnits=deg  RotationStandardAxis=+Z  RotationAngle=0.0  RotationArbitraryAxis=[0 0 1]  FollAlignAxisA=+X  BaseAlignAxisA=+Y  FollAlignAxisB=+Y  BaseAlignAxisB=+Z  RotationSequenceAxes=FollowerAxes  RotationSequence=XYZ  RotationSequenceAngles=RigKnee.rot  RotationSequenceAnglesUnits=rad  RotationMatrix=[1 0 0; 0 1 0; 0 0 1]
  RightKneeTf_B : sm_lib/Frames and Transforms/Rigid Transform  TranslationMethod=Cartesian  TranslationStandardOffset=0  TranslationLengthUnit=m  TranslationStandardAxis=+Z  TranslationCartesianOffset=RigKnee.pos  TranslationROffset=0  TranslationROffsetUnits=m  TranslationZOffset=0  TranslationZOffsetUnits=m  TranslationThetaOffset=0  TranslationThetaOffsetUnits=deg  RotationMethod=RotationSequence  RotationAngleUnits=deg  RotationStandardAxis=+Z  RotationAngle=0.0  RotationArbitraryAxis=[0 0 1]  FollAlignAxisA=+X  BaseAlignAxisA=+Y  FollAlignAxisB=+Y  BaseAlignAxisB=+Z  RotationSequenceAxes=FollowerAxes  RotationSequence=XYZ  RotationSequenceAngles=RigKnee.rot  RotationSequenceAnglesUnits=rad  RotationMatrix=[1 0 0; 0 1 0; 0 0 1]
  Scope : Scope
  Scope1 : Scope
  Mechanical connection : PMIOPort  Side=Left
  Foot sole CF : PMIOPort  Port=2  Side=Right
  Contact data : Outport
  Motor sensory data : Outport  Port=2
  Total force : Outport  Port=3
  Zero moment point : Outport  Port=4
  Leg COM-mass : Outport  Port=5
  Leg momentum : Outport  Port=6
  Leg momentum1 : Outport  Port=7
  wires:
  [T1] -> Motor1 - HipYaw/1
  [T2] -> Motor2 - HipRoll/1
  Motor1 - HipYaw/3 -> Bus Creator/3
  Motor1 - HipYaw/1 -> Bus Creator/1
  [T5] -> Motor5 - AnklePitch/1
  Motor1 - HipYaw/2 -> Bus Creator/2
  Motor2 - HipRoll/1 -> Bus Creator1/1
  Motor3_1 - HipPitch/2 -> Bus Creator2/2
  Motor2 - HipRoll/3 -> Bus Creator1/3
  Motor5 - AnklePitch/1 -> Bus Creator4/1
  Motor6 - AnkleRoll/1 -> Bus Creator5/1
  Motor5 - AnklePitch/3 -> Bus Creator4/3
  Motor5 - AnklePitch/2 -> Bus Creator4/2
  [T3_1] -> Motor3_1 - HipPitch/1
  Motor3_1 - HipPitch/4 -> Bus Creator2/4
  Motor6 - AnkleRoll/4 -> Bus Creator5/4
  Motor6 - AnkleRoll/3 -> Bus Creator5/3
  [T6] -> Motor6 - AnkleRoll/1
  Motor2 - HipRoll/2 -> Bus Creator1/2
  Motor3_1 - HipPitch/3 -> Bus Creator2/3
  Motor1 - HipYaw/4 -> Bus Creator/4
  Motor6 - AnkleRoll/2 -> Bus Creator5/2
  Motor2 - HipRoll/4 -> Bus Creator1/4
  Motor3_1 - HipPitch/1 -> Bus Creator2/1
  Motor5 - AnklePitch/4 -> Bus Creator4/4
  Bus Creator5/1 -> [Mot6]  "mot6"
  Bus Creator4/1 -> [Mot5]  "mot5"
  Bus Creator1/1 -> [Mot2]  "mot2"
  Bus Creator/1 -> [Mot1]  "mot1"
  Bus Creator2/1 -> [Mot3_1]  "mot3_1"
  Motor3_2 - HipPitch/4 -> Bus Creator7/4
  Motor3_2 - HipPitch/3 -> Bus Creator7/3
  Motor3_2 - HipPitch/1 -> Bus Creator7/1
  [T3_2] -> Motor3_2 - HipPitch/1
  Motor3_2 - HipPitch/2 -> Bus Creator7/2
  Bus Creator7/1 -> [Mot3_2]  "mot3_2"
  Motor 4_2 - KneePitch/1 -> Bus Creator8/1
  Motor 4_2 - KneePitch/4 -> Bus Creator8/4
  Bus Creator3/1 -> [Mot4_1]  "mot4_1"
  [T4_2] -> Motor 4_2 - KneePitch/1
  Motor 4_2 - KneePitch/3 -> Bus Creator8/3
  Motor 4_2 - KneePitch/2 -> Bus Creator8/2
  [T4_1] -> Motor4_1 - KneePitch/1
  Motor4_1 - KneePitch/4 -> Bus Creator3/4
  Motor4_1 - KneePitch/1 -> Bus Creator3/1
  Motor4_1 - KneePitch/3 -> Bus Creator3/3
  Motor4_1 - KneePitch/2 -> Bus Creator3/2
  Bus Creator8/1 -> [Mot4_2]  "mot4_2"
  Gain1/1 -> Gain3/1, [T4_2]
  Gain/1 -> Gain2/1, [T3_1]
  Gain2/1 -> [T3_2]
  Demux/5 -> [T5]
  Demux/1 -> [T1]
  Demux/3 -> Gain/1
  Gain3/1 -> [T4_1]
  Demux/6 -> [T6]
  Demux/4 -> Gain1/1
  Torques/1 -> Scope/1, Demux/1
  Demux/2 -> [T2]
  [Mot4_2] -> Bus Creator6/6
  [Mot3_2] -> Bus Creator6/4
  [Mot2] -> Bus Creator6/2
  Bus Creator6/1 -> Motor sensory data/1
  [Mot1] -> Bus Creator6/1
  [Mot5] -> Bus Creator6/7
  [Mot4_1] -> Bus Creator6/5
  [Mot6] -> Bus Creator6/8
  [Mot3_1] -> Bus Creator6/3
  FootContact/1 -> Bus Creator9/1
  FootContact/4 -> Bus Creator9/2
  FootContact/2 -> Total force/1
  Bus Creator9/1 -> Contact data/1
  FootContact/3 -> Zero moment point/1
  RIGHT: Link 2 dyn. ref/3 -> [FOR2]
  RIGHT: Link 6 dyn. ref/3 -> [FOR6]
  RIGHT: Link 4 dyn. ref/3 -> [FOR4]
  RIGHT: Link 5 dyn. ref/3 -> [FOR5]
  RIGHT: Link 4 dyn. ref/2 -> [MOM4]
  [FOR1] -> Add2/1
  [FOR4] -> Add2/5
  Add2/1 -> Leg momentum1/1
  [FOR2] -> Add2/2
  RIGHT: Link 3 dyn. ref/2 -> [MOM3]
  RIGHT: Link 1 dyn. ref/3 -> [FOR1]
  RIGHT: Link 3 dyn. ref/1 -> [COM3]
  [FOR3] -> Add2/4
  [COM3] -> Add/4
  [COM1] -> Add/1
  [FORD] -> Add2/3
  [MOM2] -> Add1/2
  [MOM1] -> Add1/1
  [MOM5] -> Add1/6
  RIGHT: Link 2 dyn. ref/2 -> [MOM2]
  [FOR5] -> Add2/6
  [COM5] -> Add/6
  RIGHT: Link 2 dyn. ref/1 -> [COM2]
  RIGHT: Link 6 dyn. ref/2 -> [MOM6]
  RIGHT: Link 4 dyn. ref/1 -> [COM4]
  [COM6] -> Add/7
  [COM2] -> Add/2
  RIGHT: Link 1 dyn. ref/1 -> [COM1]
  RIGHT: Link 1 dyn. ref/2 -> [MOM1]
  [COMD] -> Add/3
  RIGHT: Link 5 dyn. ref/1 -> [COM5]
  [MOM6] -> Add1/7
  RIGHT: Link 5 dyn. ref/2 -> [MOM5]
  [MOMD] -> Add1/3
  RIGHT: Link 6 dyn. ref/1 -> [COM6]
  [MOM4] -> Add1/5
  [FOR6] -> Add2/7
  Add1/1 -> Leg momentum/1
  RIGHT: Link 3 dyn. ref/3 -> [FOR3]
  Add/1 -> Leg COM-mass/1
  [COM4] -> Add/5
  [MOM3] -> Add1/4
  RightGasDamper/1 -> [COMD]
  RightGasDamper/3 -> [FORD]
  RightGasDamper/2 -> [MOMD]
  FootContact/5 -> Scope1/1
  connections:
  RightAnklePitch/RConn1 -- Motor5 - AnklePitch/LConn1
  RightAnkleRollTf/RConn1 -- Motor6 - AnkleRoll/LConn1
  Motor1 - HipYaw/LConn1 -- RightHipYawTf/RConn1
  RightHipPitchTf_1/RConn1 -- Motor3_1 - HipPitch/LConn1
  RightHipRollTf/RConn1 -- Motor2 - HipRoll/LConn1
  RightAnkleRollTf/LConn1 -- RightAnklePitchLink/RConn1 -- Motor5 - AnklePitch/RConn1
  RightHipRollTf/LConn1 -- RightHipYawLink/RConn1 -- Motor1 - HipYaw/RConn1
  RightHipPitchTf/LConn1 -- RightGasDamper/LConn1 -- Motor2 - HipRoll/RConn1 -- RightHipRollLink/RConn1
  RightHipYawTf/LConn1 -- Mechanical connection/RConn1
  RightAnkleRollLink/RConn1 -- Motor6 - AnkleRoll/RConn1 -- RightFootTf/LConn1
  RightHipPitchTf_2/RConn1 -- Motor3_2 - HipPitch/LConn1
  RightHipPitchTf/RConn1 -- RightHipPitchTf_2/LConn1 -- RightHipPitchTf_1/LConn1
  Motor4_1 - KneePitch/RConn1 -- RightKneeTf_1/LConn1
  RightKneeTf_2/RConn1 -- RightKneeTf_1/RConn1 -- RightAnklePitch/LConn1
  Motor 4_2 - KneePitch/RConn1 -- RightGasDamper/RConn1 -- RightKneeTf_2/LConn1 -- RightKneeJoint/RConn1
  Motor 4_2 - KneePitch/LConn1 -- RightKneeTf_B/RConn1
  Motor4_1 - KneePitch/LConn1 -- RightKneeTf_A/RConn1
  Motor3_2 - HipPitch/RConn1 -- RightHipPitchJoint_2/RConn1 -- RightKneeTf_B/LConn1
  Motor3_1 - HipPitch/RConn1 -- RightHipPitchJoint_1/RConn1 -- RightHipPitchDynRef/LConn1 -- RightKneeTf_A/LConn1
  FootContact/LConn1 -- RightFootTf/RConn1
  FootContact/RConn1 -- Foot sole CF/RConn1
  COM frame R3/LConn1 -- RightHipPitchDynRef/RConn1
  RIGHT: Link 1 dyn. ref/LConn1 -- RightHipYawLink/LConn1
  RIGHT: Link 2 dyn. ref/LConn1 -- RightHipRollLink/LConn1
  COM frame R3/RConn1 -- RIGHT: Link 3 dyn. ref/LConn1
  RightKneeJoint/LConn1 -- RIGHT: Link 4 dyn. ref/LConn1
  RightAnklePitchLink/LConn1 -- RIGHT: Link 5 dyn. ref/LConn1
  RIGHT: Link 6 dyn. ref/LConn1 -- RightAnkleRollLink/LConn1
